simulink model "MultiPortSwitch_2"  (R2017b)
settings: Solver=FixedStepDiscrete  StartTime=0.0  StopTime=10.0  FixedStep=0.200000  RelTol=1e-3
settings Model: Creator=hbourbou  LastModifiedBy=hbourbou
settings DataIOCC: SaveFormat=StructureWithTime
settings OptimizationCC: LifeSpan=inf
settings DebuggingCC: SFExecutionAtInitializationDiag=none
settings HardwareCC: ProdBitPerSizeT=32  ProdBitPerPtrDiffT=32  ProdWordSize=32  ProdHWDeviceType=Specified
settings CodeAppCC: StateflowObjectComments=on

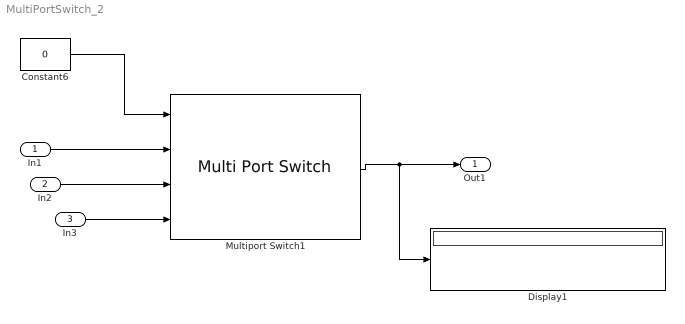
== system MultiPortSwitch_2 ==
  In1 : Inport  PortDimensions=[2,3]
  In2 : Inport  Port=2  PortDimensions=[2,3]
  In3 : Inport  Port=3  PortDimensions=[2,3]
  Constant6 : Constant  Value=0
  Display1 : Display
  Multiport Switch1 : MultiPortSwitch  DataPortOrder=Zero-based contiguous
  Out1 : Outport
  wires:
  Constant6/1 -> Multiport Switch1/1
  Multiport Switch1/1 -> Display1/1, Out1/1
  In1/1 -> Multiport Switch1/2
  In2/1 -> Multiport Switch1/3
  In3/1 -> Multiport Switch1/4
